simulink library "SimulinkLibrary"  (R2021b)
settings: Solver=VariableStepAuto  StartTime=0.0  StopTime=10.0  RelTol=1e-3
undefined symbols (not defined in the file): Ts, w0
libraries: canmsglib x6, $bdroot x5, sharedtransform x2, simulink x1
(part 3 of 3)

== stateflow chart SimulinkLibrary/Sec/CountTo60 ==
  state initialise
    entry:
    Out = 0;
  state AddOne
    entry:
    Out = Out + In;
  (default) -> initialise
  (junction 10) -> initialise
  (junction 8) -> (junction 10) : [Out >= 60]
  initialise -> AddOne : [In == 1]
  AddOne -> AddOne [order 2]
  AddOne -> (junction 8) [order 1]
  data: Out output single; In input

== matlab function SimulinkLibrary/E2E_1C_SftyInfo/SftyInfo_CalcCksm ==
  data: SftyInfo_byte3 input; cksm output; LoByte input; Nibble input; Alv_Cntr input

function cksm = CRC(SftyInfo_byte3,LoByte,Nibble, Alv_Cntr)
table = [0x00,0x1D,0x3A,0x27,0x74,0x69,0x4E,0x53,0xE8,0xF5,0xD2,0xCF,0x9C,0x81,0xA6,0xBB,0xCD,0xD0,0xF7,0xEA,0xB9,0xA4,0x83,0x9E,0x25,0x38,0x1F,0x02,0x51,0x4C,0x6B,0x76,0x87,0x9A,0xBD,0xA0,0xF3,0xEE,0xC9,0xD4,0x6F,0x72,0x55,0x48,0x1B,0x06,0x21,0x3C,0x4A,0x57,0x70,0x6D,0x3E,0x23,0x04,0x19,0xA2,0xBF,0x98,0x85,0xD6,0xCB,0xEC,0xF1,0x13,0x0E,0x29,0x34,0x67,0x7A,0x5D,0x40,0xFB,0xE6,0xC1,0xDC,0x8F,0x92,0xB5,0xA8,0xDE,0xC3,0xE4,0xF9,0xAA,0xB7,0x90,0x8D,0x36,0x2B,0x0C,0x11,0x42,0x5F,0x78,0x65,0x94,0x89,0xAE,0xB3,0xE0,0xFD,0xDA,0xC7,0x7C,0x61,0x46,0x5B,0x08,0x15,0x32,0x2F,0x59,0x44,0x63,0x7E,0x2D,0x30,0x17,0x0A,0xB1,0xAC,0x8B,0x96,0xC5,0xD8,0xFF,0xE2,0x26,0x3B,0x1C,0x01,0x52,0x4F,0x68,0x75,0xCE,0xD3,0xF4,0xE9,0xBA,0xA7,0x80,0x9D,0xEB,0xF6,0xD1,0xCC,0x9F,0x82,0xA5,0xB8,0x03,0x1E,0x39,0x24,0x77,0x6A,0x4D,0x50,0xA1,0xBC,0x9B,0x86,0xD5,0xC8,0xEF,0xF2,0x49,0x54,0x73,0x6E,0x3D,0x20,0x07,0x1A,0x6C,0x71,0x56,0x4B,0x18,0x05,0x22,0x3F,0x84,0x99,0xBE,0xA3,0xF0,0xED,0xCA,0xD7,0x35,0x28,0x0F,0x12,0x41,0x5C,0x7B,0x66,0xDD,0xC0,0xE7,0xFA,0xA9,0xB4,0x93,0x8E,0xF8,0xE5,0xC2,0xDF,0x8C,0x91,0xB6,0xAB,0x10,0x0D,0x2A,0x37,0x64,0x79,0x5E,0x43,0xB2,0xAF,0x88,0x95,0xC6,0xDB,0xFC,0xE1,0x5A,0x47,0x60,0x7D,0x2E,0x33,0x14,0x09,0x7F,0x62,0x45,0x58,0x0B,0x16,0x31,0x2C,0x97,0x8A,0xAD,0xB0,0xE3,0xFE,0xD9,0xC4];

data = zeros(1,4);
cksm = 0x00;
crc = 0x00;


data = [LoByte, 0x00 , (Nibble*0x10+Alv_Cntr), SftyInfo_byte3];


for i = 1:4
crc = table(bitxor(crc,data(i))+1);
end
crc = bitxor(crc, 0x00);

cksm = crc;

== stateflow chart SimulinkLibrary/E2E_1C_VehInfo/AliveCounter ==
  state Restart
    entry:
    Alv_Ctr = 0;
  state CountUp
    entry:
    Alv_Ctr = Alv_Ctr+1
  (default) -> Restart
  CountUp -> Restart [order 1] : [Alv_Ctr ==14]
  Restart -> CountUp
  CountUp -> CountUp [order 2]
  data: Alv_Ctr output

== matlab function SimulinkLibrary/E2E_1C_VehInfo/VehInfo_CalcCksm ==
  data: VehInfo_Byte3 input; VehInfo_Byte4 input; VehInfo_Byte5 input; VehInfo_Byte6 input; cksm output; LoByte input; Nibble input; Alv_Cntr input

function cksm = CRC(VehInfo_Byte3, VehInfo_Byte4, VehInfo_Byte5, VehInfo_Byte6,LoByte,Nibble, Alv_Cntr)
table = [0x00,0x1D,0x3A,0x27,0x74,0x69,0x4E,0x53,0xE8,0xF5,0xD2,0xCF,0x9C,0x81,0xA6,0xBB,0xCD,0xD0,0xF7,0xEA,0xB9,0xA4,0x83,0x9E,0x25,0x38,0x1F,0x02,0x51,0x4C,0x6B,0x76,0x87,0x9A,0xBD,0xA0,0xF3,0xEE,0xC9,0xD4,0x6F,0x72,0x55,0x48,0x1B,0x06,0x21,0x3C,0x4A,0x57,0x70,0x6D,0x3E,0x23,0x04,0x19,0xA2,0xBF,0x98,0x85,0xD6,0xCB,0xEC,0xF1,0x13,0x0E,0x29,0x34,0x67,0x7A,0x5D,0x40,0xFB,0xE6,0xC1,0xDC,0x8F,0x92,0xB5,0xA8,0xDE,0xC3,0xE4,0xF9,0xAA,0xB7,0x90,0x8D,0x36,0x2B,0x0C,0x11,0x42,0x5F,0x78,0x65,0x94,0x89,0xAE,0xB3,0xE0,0xFD,0xDA,0xC7,0x7C,0x61,0x46,0x5B,0x08,0x15,0x32,0x2F,0x59,0x44,0x63,0x7E,0x2D,0x30,0x17,0x0A,0xB1,0xAC,0x8B,0x96,0xC5,0xD8,0xFF,0xE2,0x26,0x3B,0x1C,0x01,0x52,0x4F,0x68,0x75,0xCE,0xD3,0xF4,0xE9,0xBA,0xA7,0x80,0x9D,0xEB,0xF6,0xD1,0xCC,0x9F,0x82,0xA5,0xB8,0x03,0x1E,0x39,0x24,0x77,0x6A,0x4D,0x50,0xA1,0xBC,0x9B,0x86,0xD5,0xC8,0xEF,0xF2,0x49,0x54,0x73,0x6E,0x3D,0x20,0x07,0x1A,0x6C,0x71,0x56,0x4B,0x18,0x05,0x22,0x3F,0x84,0x99,0xBE,0xA3,0xF0,0xED,0xCA,0xD7,0x35,0x28,0x0F,0x12,0x41,0x5C,0x7B,0x66,0xDD,0xC0,0xE7,0xFA,0xA9,0xB4,0x93,0x8E,0xF8,0xE5,0xC2,0xDF,0x8C,0x91,0xB6,0xAB,0x10,0x0D,0x2A,0x37,0x64,0x79,0x5E,0x43,0xB2,0xAF,0x88,0x95,0xC6,0xDB,0xFC,0xE1,0x5A,0x47,0x60,0x7D,0x2E,0x33,0x14,0x09,0x7F,0x62,0x45,0x58,0x0B,0x16,0x31,0x2C,0x97,0x8A,0xAD,0xB0,0xE3,0xFE,0xD9,0xC4];

data = zeros(1,7);
cksm = 0x00;
crc = 0x00;


data = [LoByte, 0x00 , (Nibble*0x10+Alv_Cntr), VehInfo_Byte3, VehInfo_Byte4, VehInfo_Byte5, VehInfo_Byte6];


for i = 1:7
crc = table(bitxor(crc,data(i))+1);
end
crc = bitxor(crc, 0x00);

cksm = crc;

== matlab function SimulinkLibrary/E2E_1C_SftyInfo/SftyInfo_CalcCksm1 ==
  data: SftyOk input; cksm output; CrashDetnNeg input; LoByte input; Nibble input; Alv_Cntr input

function cksm = CRC(SftyOk,CrashDetnNeg,LoByte,Nibble, Alv_Cntr)
table = [0x00,0x1D,0x3A,0x27,0x74,0x69,0x4E,0x53,0xE8,0xF5,0xD2,0xCF,0x9C,0x81,0xA6,0xBB,0xCD,0xD0,0xF7,0xEA,0xB9,0xA4,0x83,0x9E,0x25,0x38,0x1F,0x02,0x51,0x4C,0x6B,0x76,0x87,0x9A,0xBD,0xA0,0xF3,0xEE,0xC9,0xD4,0x6F,0x72,0x55,0x48,0x1B,0x06,0x21,0x3C,0x4A,0x57,0x70,0x6D,0x3E,0x23,0x04,0x19,0xA2,0xBF,0x98,0x85,0xD6,0xCB,0xEC,0xF1,0x13,0x0E,0x29,0x34,0x67,0x7A,0x5D,0x40,0xFB,0xE6,0xC1,0xDC,0x8F,0x92,0xB5,0xA8,0xDE,0xC3,0xE4,0xF9,0xAA,0xB7,0x90,0x8D,0x36,0x2B,0x0C,0x11,0x42,0x5F,0x78,0x65,0x94,0x89,0xAE,0xB3,0xE0,0xFD,0xDA,0xC7,0x7C,0x61,0x46,0x5B,0x08,0x15,0x32,0x2F,0x59,0x44,0x63,0x7E,0x2D,0x30,0x17,0x0A,0xB1,0xAC,0x8B,0x96,0xC5,0xD8,0xFF,0xE2,0x26,0x3B,0x1C,0x01,0x52,0x4F,0x68,0x75,0xCE,0xD3,0xF4,0xE9,0xBA,0xA7,0x80,0x9D,0xEB,0xF6,0xD1,0xCC,0x9F,0x82,0xA5,0xB8,0x03,0x1E,0x39,0x24,0x77,0x6A,0x4D,0x50,0xA1,0xBC,0x9B,0x86,0xD5,0xC8,0xEF,0xF2,0x49,0x54,0x73,0x6E,0x3D,0x20,0x07,0x1A,0x6C,0x71,0x56,0x4B,0x18,0x05,0x22,0x3F,0x84,0x99,0xBE,0xA3,0xF0,0xED,0xCA,0xD7,0x35,0x28,0x0F,0x12,0x41,0x5C,0x7B,0x66,0xDD,0xC0,0xE7,0xFA,0xA9,0xB4,0x93,0x8E,0xF8,0xE5,0xC2,0xDF,0x8C,0x91,0xB6,0xAB,0x10,0x0D,0x2A,0x37,0x64,0x79,0x5E,0x43,0xB2,0xAF,0x88,0x95,0xC6,0xDB,0xFC,0xE1,0x5A,0x47,0x60,0x7D,0x2E,0x33,0x14,0x09,0x7F,0x62,0x45,0x58,0x0B,0x16,0x31,0x2C,0x97,0x8A,0xAD,0xB0,0xE3,0xFE,0xD9,0xC4];
A = zeros(1,4);
data = zeros(1,4);
cksm = 0x00;
crc = 0x00;

A = [0,CrashDetnNeg,0,SftyOk];
% A(isspace(A)) = '';

B = 0;
for i = 1:length(A)
    B = B + (10^(i-1))*A(length(A)+1-i);
end

data = [LoByte, 0x00 , (Nibble*0x10+Alv_Cntr), 0xF0+ bin2dec(int2str(B))];


for i = 1:4
crc = table(bitxor(crc,data(i))+1);
end
crc = bitxor(crc, 0x00);

cksm = crc;

== stateflow chart SimulinkLibrary/E2E_1C_CtlCmd/AliveCounter ==
  state Restart
    entry:
    Alv_Ctr = 0;
  state CountUp
    entry:
    Alv_Ctr = Alv_Ctr+1
  (default) -> Restart
  CountUp -> Restart [order 1] : [Alv_Ctr ==14]
  Restart -> CountUp
  CountUp -> CountUp [order 2]
  data: Alv_Ctr output

== matlab function SimulinkLibrary/E2E_1C_CtlCmd/CtlCmd_CalcCksm ==
  data: VehInfo_Byte3 input; VehInfo_Byte4 input; cksm output; LoByte input; Nibble input; Alv_Cntr input

function cksm = CRC(VehInfo_Byte3, VehInfo_Byte4,LoByte,Nibble, Alv_Cntr)
table = [0x00,0x1D,0x3A,0x27,0x74,0x69,0x4E,0x53,0xE8,0xF5,0xD2,0xCF,0x9C,0x81,0xA6,0xBB,0xCD,0xD0,0xF7,0xEA,0xB9,0xA4,0x83,0x9E,0x25,0x38,0x1F,0x02,0x51,0x4C,0x6B,0x76,0x87,0x9A,0xBD,0xA0,0xF3,0xEE,0xC9,0xD4,0x6F,0x72,0x55,0x48,0x1B,0x06,0x21,0x3C,0x4A,0x57,0x70,0x6D,0x3E,0x23,0x04,0x19,0xA2,0xBF,0x98,0x85,0xD6,0xCB,0xEC,0xF1,0x13,0x0E,0x29,0x34,0x67,0x7A,0x5D,0x40,0xFB,0xE6,0xC1,0xDC,0x8F,0x92,0xB5,0xA8,0xDE,0xC3,0xE4,0xF9,0xAA,0xB7,0x90,0x8D,0x36,0x2B,0x0C,0x11,0x42,0x5F,0x78,0x65,0x94,0x89,0xAE,0xB3,0xE0,0xFD,0xDA,0xC7,0x7C,0x61,0x46,0x5B,0x08,0x15,0x32,0x2F,0x59,0x44,0x63,0x7E,0x2D,0x30,0x17,0x0A,0xB1,0xAC,0x8B,0x96,0xC5,0xD8,0xFF,0xE2,0x26,0x3B,0x1C,0x01,0x52,0x4F,0x68,0x75,0xCE,0xD3,0xF4,0xE9,0xBA,0xA7,0x80,0x9D,0xEB,0xF6,0xD1,0xCC,0x9F,0x82,0xA5,0xB8,0x03,0x1E,0x39,0x24,0x77,0x6A,0x4D,0x50,0xA1,0xBC,0x9B,0x86,0xD5,0xC8,0xEF,0xF2,0x49,0x54,0x73,0x6E,0x3D,0x20,0x07,0x1A,0x6C,0x71,0x56,0x4B,0x18,0x05,0x22,0x3F,0x84,0x99,0xBE,0xA3,0xF0,0xED,0xCA,0xD7,0x35,0x28,0x0F,0x12,0x41,0x5C,0x7B,0x66,0xDD,0xC0,0xE7,0xFA,0xA9,0xB4,0x93,0x8E,0xF8,0xE5,0xC2,0xDF,0x8C,0x91,0xB6,0xAB,0x10,0x0D,0x2A,0x37,0x64,0x79,0x5E,0x43,0xB2,0xAF,0x88,0x95,0xC6,0xDB,0xFC,0xE1,0x5A,0x47,0x60,0x7D,0x2E,0x33,0x14,0x09,0x7F,0x62,0x45,0x58,0x0B,0x16,0x31,0x2C,0x97,0x8A,0xAD,0xB0,0xE3,0xFE,0xD9,0xC4];

data = zeros(1,5);
cksm = 0x00;
crc = 0x00;


data = [LoByte, 0x00 , (Nibble*0x10+Alv_Cntr), VehInfo_Byte3, VehInfo_Byte4];


for i = 1:5
crc = table(bitxor(crc,data(i))+1);
end
crc = bitxor(crc, 0x00);

cksm = crc;

== stateflow chart SimulinkLibrary/ErrDetDelay ==
  state No_error
    entry:
    Err_B_Detd = boolean(0);
  state Error_Det_Review
    entry:
    Err_B_Detd = boolean(0);
  state Error_Confirmed
    entry:
    Err_B_Detd = boolean(1);
  (default) -> No_error
  (junction 11) -> No_error
  (junction 9) -> (junction 11) : [ErrCdn == 0]
  No_error -> Error_Det_Review : [ErrCdn == 1] % Error condition is true
  Error_Det_Review -> (junction 9) [order 1]
  (junction 25) -> (junction 9)
  Error_Det_Review -> Error_Confirmed [order 2] : [after (DetnDly, sec)] % Detction delay
  Error_Confirmed -> (junction 25)
  data: Err_B_Detd output; ErrCdn input; DetnDly input

== stateflow chart SimulinkLibrary/Bundles/HwSelProc/Chart ==
  state Heal
    entry:
    Out = 0;
  state ReadyToTrigger
    entry:
    Out = 0;
  state ReadyToHeal
    entry:
    Out = 1;
  state Trigger
    entry:
    Out = 1;
  (default) -> Heal
  Heal -> ReadyToTrigger : [In==1]
  ReadyToTrigger -> Heal [order 1] : [In==0]
  ReadyToHeal -> Heal [order 1] : [after(HealTime,sec)]
  ReadyToTrigger -> Trigger [order 2] : [after(TriggerTime,sec)]
  ReadyToHeal -> Trigger [order 2] : [In==1]
  Trigger -> ReadyToHeal : [In==0]
  data: In input; HealTime input; TriggerTime input; Out output

== stateflow chart SimulinkLibrary/Debounce ==
  state Heal
    entry:
    Out = 0;
  state ReadyToTrigger
    entry:
    Out = 0;
  state ReadyToHeal
    entry:
    Out = 1;
  state Trigger
    entry:
    Out = 1;
  (default) -> Heal
  Heal -> ReadyToTrigger : [In==1]
  ReadyToTrigger -> Heal [order 1] : [In==0]
  ReadyToHeal -> Heal [order 1] : [after(HealTime,sec)]
  ReadyToTrigger -> Trigger [order 2] : [after(TriggerTime,sec)]
  ReadyToHeal -> Trigger [order 2] : [In==1]
  Trigger -> ReadyToHeal : [In==0]
  data: In input; HealTime input; TriggerTime input; Out output

== stateflow chart SimulinkLibrary/Bundles/HwSelProc/Chart1 ==
  state Heal
    entry:
    Out = 0;
  state ReadyToTrigger
    entry:
    Out = 0;
  state ReadyToHeal
    entry:
    Out = 1;
  state Trigger
    entry:
    Out = 1;
  (default) -> Heal
  Heal -> ReadyToTrigger : [In==1]
  ReadyToTrigger -> Heal [order 1] : [In==0]
  ReadyToHeal -> Heal [order 1] : [after(HealTime,sec)]
  ReadyToTrigger -> Trigger [order 2] : [after(TriggerTime,sec)]
  ReadyToHeal -> Trigger [order 2] : [In==1]
  Trigger -> ReadyToHeal : [In==0]
  data: In input; HealTime input; TriggerTime input; Out output

== stateflow chart SimulinkLibrary/Bundles/HwSelProc/Chart2 ==
  state Heal
    entry:
    Out = 0;
  state ReadyToTrigger
    entry:
    Out = 0;
  state ReadyToHeal
    entry:
    Out = 1;
  state Trigger
    entry:
    Out = 1;
  (default) -> Heal
  Heal -> ReadyToTrigger : [In==1]
  ReadyToTrigger -> Heal [order 1] : [In==0]
  ReadyToHeal -> Heal [order 1] : [after(HealTime,sec)]
  ReadyToTrigger -> Trigger [order 2] : [after(TriggerTime,sec)]
  ReadyToHeal -> Trigger [order 2] : [In==1]
  Trigger -> ReadyToHeal : [In==0]
  data: In input; HealTime input; TriggerTime input; Out output

== stateflow chart SimulinkLibrary/CountUp ==
  state initialise
    entry:
    Out = 0;
  state AddOne
    entry:
    Out = (Out + 1);
  (default) -> initialise
  (junction 10) -> initialise
  (junction 8) -> (junction 10) : [after (1,sec)]
  initialise -> AddOne : [after (1,sec)]
  AddOne -> AddOne [order 2] : [after(1,sec)]
  AddOne -> (junction 8) [order 1] : [Out >= MaxVal]
  data: Out output uint8; MaxVal input

== stateflow chart SimulinkLibrary/Bundles/HwSelProc/Chart3 ==
  state Neutral
    entry:
    DMS_HwEltGearPosn_Zs = 0;
  state Reverse
    entry:
    DMS_HwEltGearPosn_Zs = 2;
  state Drive
    entry:
    DMS_HwEltGearPosn_Zs = 1;
  (default) -> Neutral
  Neutral -> Drive [order 1] : [
      | DrvBtn_B_PsdFild ...
      | && DMS_GearLock_B_Reqd ==0;
      | ]
  Drive -> Neutral [order 1] : [NeutBtn_B_PsdFild]
  Reverse -> Neutral [order 1] : [NeutBtn_B_PsdFild]
  Neutral -> Reverse [order 2] : [
      | RvrsBtn_B_PsdFild ...
      | && DMS_GearLock_B_Reqd ==0;
      | ]
  Reverse -> Drive [order 2] : [
      | DrvBtn_B_PsdFild ...
      | && DMS_GearLock_B_Reqd ==0;
      | ]
  Drive -> Reverse [order 2] : [
      | RvrsBtn_B_PsdFild ...
      | && DMS_GearLock_B_Reqd ==0;
      | ]
  data: DMS_HwEltGearPosn_Zs output; DrvBtn_B_PsdFild input; RvrsBtn_B_PsdFild input; NeutBtn_B_PsdFild input; DMS_GearLock_B_Reqd input

== stateflow chart SimulinkLibrary/HiDelay ==
  state Lo
    entry:
    Sig_Out = boolean(0)
  state Hi
    entry:
    Sig_Out = boolean(1)
  (default) -> Lo
  Hi -> Lo : [Sig_In == 0]
  Lo -> Hi : [duration(Sig_In ==1) >= Delay_T_Z]
  data: Sig_Out output boolean; Sig_In input boolean; Delay_T_Z input

== stateflow chart SimulinkLibrary/Scheduler(10ms base) ==
  note: This is a simple scheduler using
      | temporal logic and output events E1,E2
  state SynchronousScheduler [parallel]
    % 10ms rate
    on every(1,'tick'): send(E10ms);
    % 100ms rate
    on every(10,'tick'): send(E100ms);
    settings: executionOrder=1
  events: E10ms output FUNCTION_CALL_EVENT; E100ms output FUNCTION_CALL_EVENT

== stateflow chart SimulinkLibrary/ErrDetDelayResetOvrrd ==
  state No_error
    entry:
    Err_B_Detd = boolean(0);
  state Error_Det_Review
    entry:
    Err_B_Detd = boolean(0);
  state Error_Confirmed
    entry:
    Err_B_Detd = boolean(1);
  (default) -> No_error
  (junction 11) -> No_error
  (junction 35) -> No_error
  (junction 9) -> (junction 11) : [ErrCdn == 0]
  (junction 39) -> (junction 35) : [Reset_B]
  No_error -> Error_Det_Review : [ErrCdn == 1] % Error condition is true
  Error_Det_Review -> (junction 9) [order 1]
  Error_Det_Review -> (junction 39) [order 3]
  (junction 25) -> (junction 9)
  (junction 31) -> (junction 39)
  Error_Det_Review -> (junction 20) [order 2] : [after (DetnDly_T, sec)] % Detction delay
  (junction 20) -> Error_Confirmed : [ErrCdn == 1 ]
  Error_Confirmed -> (junction 25) [order 1]
  Error_Confirmed -> (junction 31) [order 2]
  data: Err_B_Detd output; ErrCdn input; Reset_B input; DetnDly_T input

== stateflow chart SimulinkLibrary/TimerStartStop ==
  state initialise
    entry:
    Timer_T = 0;
  state AddOne
    entry:
    Timer_T = (Timer_T + 1);
  (default) -> initialise
  (junction 3) -> initialise
  (junction 9) -> (junction 3) : [after (1,sec)]
  initialise -> (junction 16) : [Count_B_Ena]
  (junction 16) -> AddOne : [after (1,sec)]
  AddOne -> AddOne [order 2] : [after(1,sec)]
  AddOne -> (junction 9) [order 1] : [Count_B_Ena==0]
  data: Count_B_Ena input; Timer_T output double

== stateflow chart SimulinkLibrary/CountUp_SampleBased ==
  state initialise
    entry:
    Out = 0;
  state AddOne
    entry:
    Out = (Out + 1);
  (default) -> initialise
  (junction 10) -> initialise
  (junction 8) -> (junction 10)
  initialise -> AddOne
  AddOne -> AddOne [order 2]
  AddOne -> (junction 8) [order 1] : [Out >= MaxVal]
  data: Out output uint8; MaxVal input

== stateflow chart SimulinkLibrary/FaultDetect ==
  state Fault_Inactive
    entry:
    Flt_B_Acvd = boolean(0);
  state Evaluate
  state Fault_Active
    entry:
    Flt_B_Acvd = boolean(1);
  (default) -> Fault_Inactive
  (junction 11) -> Fault_Inactive
  (junction 9) -> (junction 11) : [FltCdn_B_Detd == boolean(0) ] % fault not detected
  Fault_Active -> Fault_Inactive : [
      | FltCdn_B_Detd == boolean(0)...
      | && Flt_B_Rst == boolean(1) % Fault reset requested
      | ]
  Fault_Inactive -> (junction 15) : [FltCdn_B_Detd]
  (junction 15) -> Evaluate : [after(FltDetn_Tms, msec)]
  Evaluate -> (junction 9) [order 1]
  Evaluate -> Fault_Active [order 2] : %Fault still present
  data: FltCdn_B_Detd input; Flt_B_Acvd output; Flt_B_Rst input; FltDetn_Tms input

== stateflow chart SimulinkLibrary/CountUp_SampleBased_WithReset ==
  state initialise
    entry:
    Out = 0;
  state AddOne
    entry:
    Out = (Out + 1);
  (default) -> initialise
  (junction 10) -> initialise
  (junction 8) -> (junction 10)
  initialise -> AddOne : [Reset_B ==0]
  AddOne -> AddOne [order 2]
  AddOne -> (junction 8) [order 1] : [Reset_B]
  data: Out output uint8; Reset_B input

== stateflow chart SimulinkLibrary/E2E_1C_SftyInfo/AliveCounter ==
  state Restart
    entry:
    Alv_Ctr = 0;
  state CountUp
    entry:
    Alv_Ctr = Alv_Ctr+1
  (default) -> Restart
  CountUp -> Restart [order 1] : [Alv_Ctr ==14]
  Restart -> CountUp
  CountUp -> CountUp [order 2]
  data: Alv_Ctr output

== matlab function SimulinkLibrary/DiscreteSecondOrderSection/MATLAB Function ==
  data: w input; a output; zeta input; tau input; b output; c output
function [a,b,c] = fcn(w,zeta,tau)
% Formulas for Tustin discretization of w^2/(s^2 + 2*zeta*w*s + s^2)
%#codegen
wt = tau*w;    % w*tau
p = 2*zeta*wt;
q = wt^2;
r = 1+q;
d = p+r;
a = q/d;       % wt^2/(1+2*zeta*wt+wt^2)
b = (1-q)/d;   % (1-wt^2)/(1+2*zeta*wt+wt^2)
c = (r-p)/d;   % (1-2*zeta*wt+wt^2)/(1+2*zeta*wt+wt^2)
